simulink model "RStanu"  (R2018b)
settings: Solver=FixedStepAuto  StartTime=0.0  StopTime=5000  FixedStep=10  RelTol=1e-3
values from neighbouring files (symbols this model uses):
  A = [((-1 * Cp0) - k1 - kp)/CVw, kp/CVw; kp/CVp, (-kp-k2)/CVp]    [script1.m]
  B = [Cp0/CVw, k1/CVw, 0; 0, 0, k2/CVp]    [script1.m]
  C = [1, 0; 0, 1]    [script1.m]
  D = [0, 0, 0; 0, 0, 0]    [script1.m]
  dt = 500    [script1.m]
  dTg = 0    [script1.m]
  dTkz = -2    [script1.m]
  dTzew = 0    [script1.m]
  E = [Twew0, Tp0]    [script1.m]
  Tg0 = TgN    (= -10)    [script1.m]
  Tkz0 = TkzN + 2    (= 37)    [script1.m]
  Tzew0 = TzewN    (= -20)    [script1.m]
settings Model: Creator=wojciechkonury  LastModifiedBy=wojciechkonury

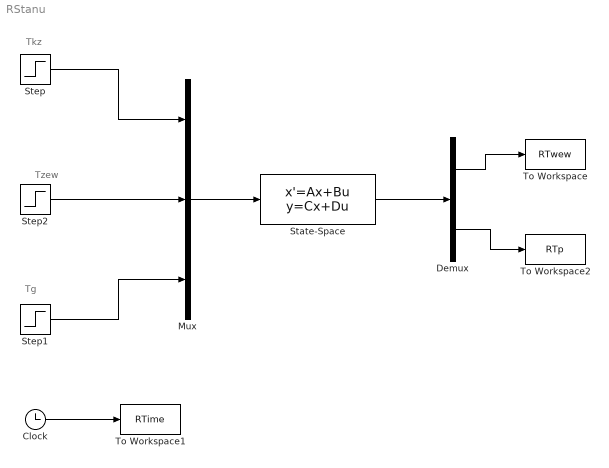
== system RStanu ==
  note: Tg
  note: Tzew
  note: Tkz
  Clock : Clock
  Demux : Demux  Outputs=2
  Mux : Mux  Inputs=3
  State-Space : StateSpace  A=A  B=B  C=C  D=D  InitialCondition=E
  Step : Step  Time=dt  Before=Tkz0  After=Tkz0 + dTkz  SampleTime=0
  Step1 : Step  Time=dt  Before=Tg0  After=Tg0 + dTg  SampleTime=0
  Step2 : Step  Time=dt  Before=Tzew0  After=Tzew0 + dTzew  SampleTime=0
  To Workspace : ToWorkspace  VariableName=RTwew  SampleTime=-1
  To Workspace1 : ToWorkspace  VariableName=RTime  SampleTime=-1
  To Workspace2 : ToWorkspace  VariableName=RTp  SampleTime=-1
  wires:
  Step1/1 -> Mux/3
  Step2/1 -> Mux/2
  Step/1 -> Mux/1
  Mux/1 -> State-Space/1
  State-Space/1 -> Demux/1
  Demux/2 -> To Workspace2/1
  Demux/1 -> To Workspace/1
  Clock/1 -> To Workspace1/1
